simulink model "Controller"  (R2020b)
settings: Solver=VariableStepAuto  StartTime=0.0  StopTime=100  RelTol=1e-3
values from neighbouring files (symbols this model uses):
  Ki = 40.0    [CruiseControlData.sldd]
  Kp = 800.0    [CruiseControlData.sldd]
settings Model: DataDictionary=CruiseControlData.sldd  Creator=Pavan  LastModifiedBy=Pavan
settings DataIOCC: SaveOutput=off  SaveTime=off

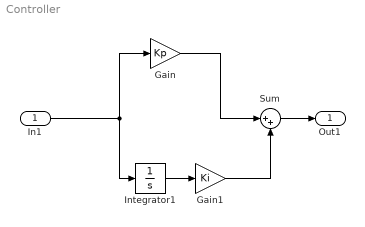
== system Controller ==
  In1 : Inport  OutDataTypeStr=double  PortDimensions=1  SampleTime=0
  Gain : Gain  Gain=Kp
  Gain1 : Gain  Gain=Ki
  Integrator1 : Integrator
  Sum : Sum  Inputs=|++
  Out1 : Outport  OutDataTypeStr=double  PortDimensions=1  SampleTime=0
  wires:
  Integrator1/1 -> Gain1/1
  Gain/1 -> Sum/1
  Gain1/1 -> Sum/2
  In1/1 -> Gain/1, Integrator1/1
  Sum/1 -> Out1/1
